simulink model "test1_aquad"  (R2016a)
settings: Solver=VariableStepAuto  StartTime=0.0  StopTime=10.0  RelTol=1e-3
settings Model: Creator=ridhi  LastModifiedBy=ridhi

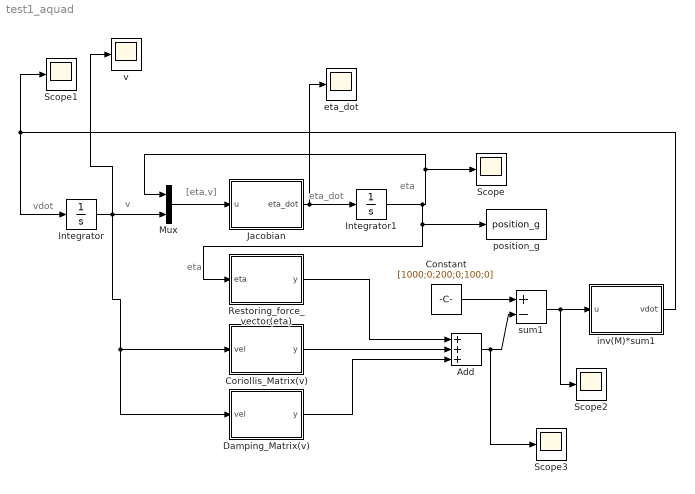
== system test1_aquad ==
  note: vdot
  note: eta
  note: v
  note: eta
  note: eta_dot
  note: [eta,v]
  Add : Sum  Inputs=+++
  Constant : Constant  Value=[1000;0;200;0;100;0]
  Coriollis_Matrix(v) : MATLAB Function  TreatAsAtomicUnit=on
  Damping_Matrix(v) : MATLAB Function  TreatAsAtomicUnit=on
  Integrator : Integrator  InitialCondition=[0;0;0;0;0;0]
  Integrator1 : Integrator  InitialCondition=[0;0;0;0;0;0]  LimitOutput=on
  Jacobian : MATLAB Function  TreatAsAtomicUnit=on
  Mux : Mux  Inputs=2
  Restoring_force_vector(eta) : MATLAB Function  TreatAsAtomicUnit=on
  Scope{,1..3} (4 alike) : Scope
  eta_dot : Scope
  inv(M)*sum1 : MATLAB Function  TreatAsAtomicUnit=on
  position_g : ToWorkspace  VariableName=position_g  SaveFormat=Timeseries  SampleTime=-1
  sum1 : Sum  Inputs=+-
  "v " : Scope
  wires:
  Integrator/1 -> "v "/1, Mux/2, Damping_Matrix(v)/1(vel), Coriollis_Matrix(v)/1(vel)
  Mux/1 -> Jacobian/1(u)
  Jacobian/1(eta_dot) -> eta_dot/1, Integrator1/1
  Integrator1/1 -> position_g/1, Restoring_force_vector(eta)/1(eta), Scope/1, Mux/1
  Restoring_force_vector(eta)/1(y) -> Add/1
  Coriollis_Matrix(v)/1(y) -> Add/2
  Damping_Matrix(v)/1(y) -> Add/3
  Add/1 -> Scope3/1, sum1/2
  inv(M)*sum1/1(vdot) -> Integrator/1, Scope1/1
  sum1/1 -> Scope2/1, inv(M)*sum1/1(u)
  Constant/1 -> sum1/1

== matlab function test1_aquad/Coriollis_Matrix(v) ==
  data: vel input; y output
function y = fcn(vel)
u = vel(1);
v = vel(2);
w = vel(3);
p = vel(4);
q = vel(5);
r = vel(6);



C_rb=[0                0           0           0           32.16*q+1462*w  32.16*r-1462*v;
       0                0           0           -1462*w     -32.16*p        1462*u;
       0                0           0           1462*v      -1462*u         -32.16*p;
       0                1462*w      -1462*v     0           2848.97*r       -1850.34*q;
       -32.16*q-1462*w  32.16*p     1462*u      -2848.97*r  0               498.63*p;
       -32.16*r+1462*v  -1462*u     32.16*p     1850.34*q   -498.63*p       0];
 
C_a= [0                     0                       0                       0                       7040.36*w-277.20*q      -1049.21*v+996.04*r;
      0                     0                       0                       -7040.36*w+277.20*q     0                       323.10*u;
      0                     0                       0                       1049.21*v-996.04*r       -323.10*u               0;
      0                     7040.36*w-277.20*q      -1049.21*v+996.04*r     0                       -996.04*v+8584.25*r     -277.20*w+7045.28*q;
      -7040.36*w+277.20*q   0                       323.10*u                996.04*v-8584.25*r      0                       645.85*p;
      1049.21*v-996.04*r    -323.10*u               0                       -277.20*w+7045.28*q     -645.85*p               0];

C = C_rb+C_a;
y = C*vel;
end

== matlab function test1_aquad/Jacobian ==
  data: u input; eta_dot output
function eta_dot = fcn(u)

v = u(7:12); %body_frame_velocities

phi=u(4); %roll
theta=u(5); %pitch
si=u(6);   %yaw
c_p=cos(phi);
c_t=cos(theta);
c_s=cos(si);
s_p=sin(phi);
s_t=sin(theta);
s_s=sin(si);
t_t=tan(theta);


J1=[c_s*c_t    -s_s*c_p+s_p*s_t*c_s     s_s*s_p+s_t*c_s*c_p;
    s_s*c_t     c_s*c_p+s_p*s_t*s_s    -c_s*s_p+s_t*s_s*c_p;
     -s_t            s_p*c_t                 c_p*c_t       ];
       
J2=[1      s_p*t_t     c_p*t_t;
    0        c_p        -s_p;
    0      s_p/c_t     c_p/c_t ];


J=[J1 zeros(3,3); zeros(3,3) J2];
eta_dot = J * v; % y == earth_velocities

end

== matlab function test1_aquad/Damping_Matrix(v) ==
  data: vel input; y output
function y = fcn(vel)
u = vel(1);
v = vel(2);
w = vel(3);
p = vel(4);
q = vel(5);
r = vel(6);
D=  [13.62+32.29*abs(u) -17.20-22.58*abs(v)     28.26+607.6*abs(w)      0       0       0;
     0                  534.9+607.6*abs(v)      0                       0       0       -1381.55;
     0                  0                       1441.25+2859.41*abs(w)  0       2052.86 0;
     0                  0                       0                       2050.3  0       0;
     0                  0                       -3105.27+381.04*abs(w)  0       6497.65 0;
     0                  372.11-1006.48*abs(v)   0                       0       0       1194.31];

y = D*vel;
end

== matlab function test1_aquad/Restoring_force_vector(eta) ==
  data: eta input; y output
function y = fcn(eta)

theta = eta(5);
phi = eta(4);

G=   [-49*sin(theta);
       49*cos(theta)*sin(phi);
       49*cos(theta)*cos(phi);
       215.87*cos(theta)*sin(phi);
       215.87*sin(theta)-1.1*cos(theta)*cos(phi);
       1.1*cos(theta)*sin(phi)];
y =  G;

end

== matlab function test1_aquad/inv(M)*sum1 ==
  data: u input; vdot output
function vdot = fcn(u)
sum1 = u;

M_rb=[1462  0      0     0       0        0;
      0     1462   0     0       0        -32.16;
      0     0      1462  0       32.16    0;
      0     0      0     498.63  0        0;
      0     0      32.16 0       1850.34  0;
      0     -32.16 0     0       0        2348.97];
  
M_a=[323.10 0       0       0       0       0;
     0      1049.21 0       0       0       -999.04;
     0      0       7040.36 0       -277.20 0;
     0      0       0       645.85  0       0;
     0      0       -277.20 0       7045.28 0;
     0      -996.04 0       0       0       8584.25];
 
M=M_rb+M_a; 

vdot = inv(M)*sum1;

end
